simulink model "Lab5_ConstantFeedback"  (R2016a)
settings: Solver=VariableStepAuto  StartTime=0.0  StopTime=30  RelTol=1e-3
settings Model: Creator=jordan  LastModifiedBy=jordan

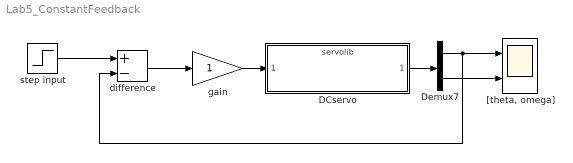
== system Lab5_ConstantFeedback ==
  DCservo : ModelReference  ModelNameDialog=servolib.slx  SimulationMode=Normal  ModelReferenceVersion=1.18
  Demux7 : Demux  Outputs=2
  "[theta, omega]" : Scope  NumInputPorts=2
  difference : Sum  Inputs=+-
  gain : Gain
  step input : Step  After=10  SampleTime=0
  wires:
  Demux7/2 -> "[theta, omega]"/2
  step input/1 -> difference/1
  difference/1 -> gain/1
  DCservo/1 -> Demux7/1
  Demux7/1 -> difference/2, "[theta, omega]"/1
  gain/1 -> DCservo/1
